simulink model "DataGeneration_ToDB"  (R2017b)
settings: Solver=ode5  StartTime=0.0  StopTime=85500  FixedStep=0.0025  RelTol=1e-3  AbsTol=1e-6
libraries: DABLib x1
settings Model: Creator=weste  LastModifiedBy=weste
settings DataIOCC: SaveFormat=Array  SignalLoggingSaveFormat=ModelDataLogs
settings OptimizationCC: BlockReduction=off  BooleanDataType=off
settings DebuggingCC: SaveWithParameterizedLinksMsg=none  UnderspecifiedInitializationDetection=Classic  MergeDetectMultiDrivingBlocksExec=none  SignalResolutionControl=TryResolveAllWithWarning  MultiTaskDSMMsg=warning  MultiTaskCondExecSysMsg=none
settings HardwareCC: TargetUnknown=on
settings ModelReferenceCC: PropagateSignalLabelsOutOfModel=off
settings GRTTargetCC: TargetLangStandard=C89/C90 (ANSI)  CombineOutputUpdateFcns=off  GRTInterface=on

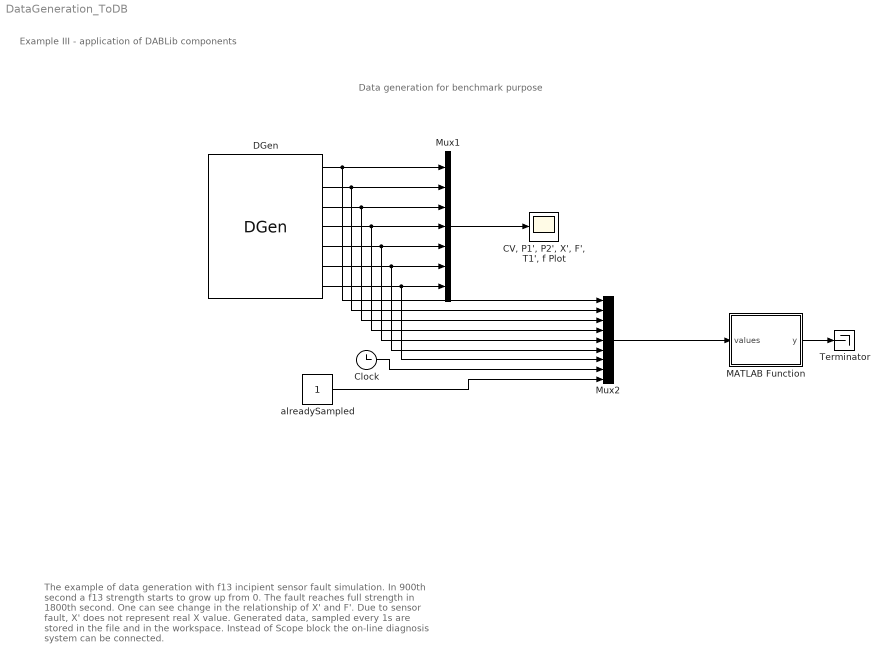
== system DataGeneration_ToDB ==
  note: Data generation for benchmark purpose
  note: Example III - application of DABLib components
  note: The example of data generation with f13 incipient sensor fault simulation.
      | In 900th second a f13 strength starts to grow up from 0.
      | The fault reaches full strength in 1800th second.
      | One can see change in the relationship of X' and F'.
      | Due to sensor fault, X' does not represent real X value.
      | Generated data, sampled every 1s are stored in the file and in the workspace.
      | Instead of Scope block the on-line diagnosis system can be connected.
  "CV, P1', P2', X', F', T1', f Plot" : Scope
  Clock : Clock
  DGen : DABLib/DGen  FSel=f13 - Rod displacement sensor fault  FType=Incipient
  MATLAB Function : MATLAB Function  TreatAsAtomicUnit=on
  Mux1 : Mux  Inputs=7
  Mux2 : Mux  Inputs=9
  Terminator : Terminator
  alreadySampled : Constant  VectorParams1D=off
  wires:
  Mux1/1 -> "CV, P1', P2', X', F', T1', f Plot"/1
  DGen/7 -> Mux2/7, Mux1/7
  DGen/6 -> Mux2/6, Mux1/6
  DGen/5 -> Mux1/5, Mux2/5
  DGen/3 -> Mux2/3, Mux1/3
  DGen/2 -> Mux2/2, Mux1/2
  DGen/1 -> Mux1/1, Mux2/1
  DGen/4 -> Mux1/4, Mux2/4
  Mux2/1 -> MATLAB Function/1(values)
  Clock/1 -> Mux2/8
  alreadySampled/1 -> Mux2/9
  MATLAB Function/1(y) -> Terminator/1

== matlab function DataGeneration_ToDB/MATLAB Function ==
  data: values input; y output
function y = saveToDB(values)

coder.extrinsic('set_param');
coder.extrinsic('evalin');
coder.extrinsic('disp');

alreadySampled = values(9);
time = values(8);

intTime=floor(time);
fracTime=time-intTime;

%Write samples to the database
if fracTime == 0 && mod(intTime,5) == 0 && alreadySampled == 0
    set_param('DataGeneration_toDB/alreadySampled', 'Value', '1');
    alreadySampled = 1;
    conn = evalin('base', 'dbconn');
    writeToDB(conn, values(1:8));
elseif alreadySampled == 1 && mod(intTime,5) ~= 0
    set_param('DataGeneration_toDB/alreadySampled', 'Value', '0');
    alreadySampled = 0;
end

y = alreadySampled;

end

function writeToDB(dbConn, values)

    coder.extrinsic('evalin');
    coder.extrinsic('sprintf');
    coder.extrinsic('datestr');
    coder.extrinsic('exec');

    controlValue = values(1);
    pressureValveInlet = values(2);
    pressureValveOutlet = values(3);
    rodDisplacement = values(4);
    disturbedMediumFlow = values(5);
    mediumTemperature = values(6);
    faultIntensity = values(7);
    elapsedSecond = values(8);
   
    startDateTime = evalin('base', 'today');
    
    currentDateTime = updateDateTime(startDateTime, elapsedSecond);
    
    %fastinsert(dbConn,'valveReadings', colNames, insertdata)
    
    query = sprintf("INSERT INTO valveReadings(timestamp, externalControllerOutput, disturbedMediumFlow, "+...
    "pressureValveInlet, pressureValveOutlet, mediumTemperature, rodDisplacement, faultIntensity)"+ ...
    "VALUES ('%s', %f, %f, %f, %f, %f, %f, %f);", datestr(currentDateTime, 'yyyy-mm-dd HH:MM:SS'), ...
    controlValue, disturbedMediumFlow, pressureValveInlet, pressureValveOutlet, mediumTemperature, ...
    rodDisplacement, faultIntensity);
    curs = exec(dbConn, query);
    disp(curs);
    
    %query = sprintf("INSERT INTO valveReadings(timestamp, externalControllerOutput, undisturbedMediumFlow, "+...
    %"pressureValveInlet, pressureValveOutlet, mediumTemperature, rodDisplacement, disturbedMediumFlow) VALUES ('%s', %f, %f, %f," + ...  
    %" %f, %f, %f, %f);", datestr(currentDateTime, 'yyyy-mm-dd HH:MM:SS'), externalControllerOutput, undisturbedMediumFlow, pressureValveInlet, ...
    %pressureValveOutlet, mediumTemperature, rodDisplacement, disturbedMediumFlow);

end

function currentDateTime = updateDateTime(startDateTime, elapsedSeconds)

    coder.extrinsic('datetime');

    hours = 0;
    minutes = 0;
    seconds = 0;

    days = fix(elapsedSeconds/86400);
    reminder = mod(elapsedSeconds,86400);
    
    if reminder ~= 0
        
        hours = fix(reminder/3600);
        reminder = mod(reminder,3600);
        
        if reminder ~= 0
            minutes = fix(reminder/60);
            seconds = mod(reminder,60);
        end
        
    end
    
    currentDateTime = datetime(2017, 10, days, hours, minutes, seconds, 0);

end
